simulink model "E010A5_R3_E1_event_queue_alloc_40A_1A_20260701_085331"  (R2024b)
settings: Solver=VariableStepAuto  StartTime=0.0  StopTime=0.54e-3  MaxStep=5e-9  RelTol=1e-3
undefined symbols (not defined in the file): A_init, A_lower, A_upper, Cout, DCR_L1, DCR_L2, DCR_L3, DCR_L4, E010_AreaBleed_Enable, E010_AreaHold_Enable, E010_AreaHold_Time, E010_PulseInhibit_Count, E010_PulseInhibit_Enable, E010_PulseInhibit_Time, E010_Reentry_Band_Down, E010_ReentryGuard_Enable, E010_TonTrunc_Enable, E010_Vref, E010A5_DeltaI_Drop_Threshold_High, E010A5_IL_Sense_Gain1, E010A5_IL_Sense_Gain2, E010A5_IL_Sense_Gain3, E010A5_IL_Sense_Gain4, E010A5_R3_AreaIntReentryTarget, E010A5_R3_AreaIntRestoreRate, E010A5_R3_AreaQueueCouplingEnable, E010A5_R3_EventQueue_Enable, E010A5_R3_FirstTonLimit, E010A5_R3_QueueMaxDepth, E010A5_R3_QueueReleaseMaxPerWindow, E010A5_R3_QueueReleaseMinSpacing, E010A5_R3_QueueSpacingEnable, E010A5_R3_TonBudget, E010A5_R3_TonBudgetWindow, E010A5_R3_TonMinMeaningful, E010A5_R3_TonRampMax, E010A5_R3_TonRampStep, E010A5_R3_UndershootBudget, E010A5_R3_UpperReentryBand, E010A5_R3_VoltageWindowEnable, ESR_C, IdealIQCOT_Enable, IL_adc_counts_per_A, IL_pk_limit_adc_neg, IL_pk_limit_adc_pos, Iload_final, Iload_initial, Iph, Iqcot_enable, kappa_cmd, Kiqcot, Kvc_iqcot, L, Lambda0_iqcot, Lambda_m2, rho_cmd, Ri_iqcot, t_load_step, Tblank, Tdead ... (+17)
libraries: simulink x29, spsCurrentMeasurementLib x8, spsMosfetLib x8, spsSeriesRLCBranchLib x5, spsVoltageMeasurementLib x5, spsDCVoltageSourceLib x4, spsControlledCurrentSourceLib x1, spsGroundLib x1, spspowerguiLib x1
(part 2 of 2)

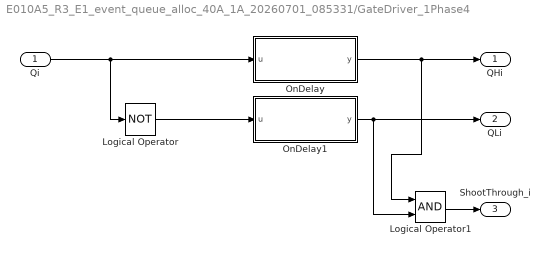
== system E010A5_R3_E1_event_queue_alloc_40A_1A_20260701_085331/GateDriver_1Phase4 ==
  Qi : Inport
  Logical Operator : Logic  Operator=NOT  AllPortsSameDT=off  OutDataTypeStr=boolean
  Logical Operator1 : Logic  AllPortsSameDT=off  OutDataTypeStr=boolean
  OnDelay : Subsystem
  OnDelay1 : Subsystem
  QHi : Outport
  QLi : Outport  Port=2
  ShootThrough_i : Outport  Port=3
  wires:
  Qi/1 -> Logical Operator/1, OnDelay/1(u)
  OnDelay/1(y) -> Logical Operator1/1, QHi/1
  Logical Operator/1 -> OnDelay1/1(u)
  OnDelay1/1(y) -> QLi/1, Logical Operator1/2
  Logical Operator1/1 -> ShootThrough_i/1

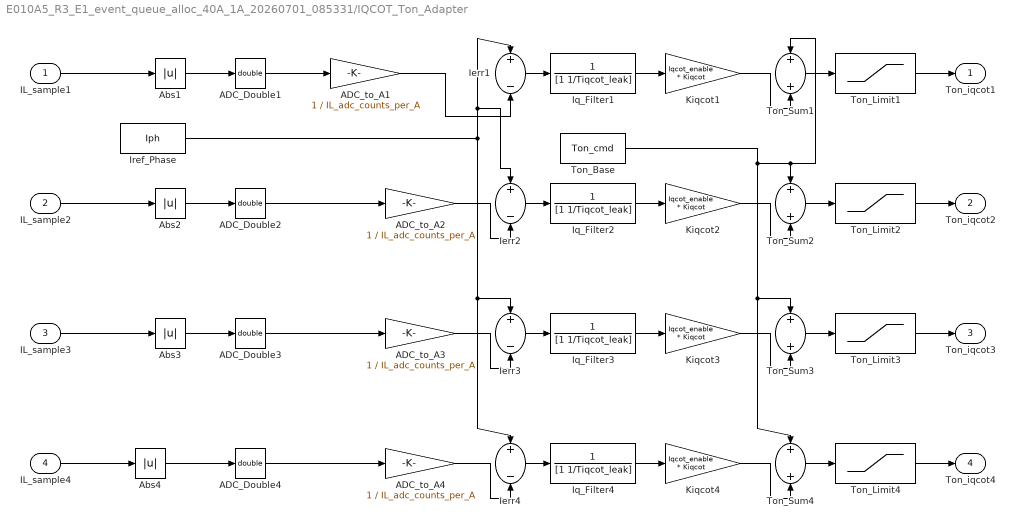
== system E010A5_R3_E1_event_queue_alloc_40A_1A_20260701_085331/IQCOT_Ton_Adapter ==
  IL_sample1 : Inport
  IL_sample2 : Inport  Port=2
  IL_sample3 : Inport  Port=3
  IL_sample4 : Inport  Port=4
  ADC_Double{1..4} (4 alike) : DataTypeConversion  OutDataTypeStr=double  SaturateOnIntegerOverflow=off  RndMeth=Floor
  ADC_to_A{1..4} (4 alike) : Gain  Gain=1 / IL_adc_counts_per_A  OutDataTypeStr=double
  Abs{1..4} (4 alike) : Abs  SaturateOnIntegerOverflow=off
  Ierr{1..4} (4 alike) : Sum  Inputs=+-
  Iq_Filter{1..4} (4 alike) : TransferFcn  Numerator=1  Denominator=[1 1/Tiqcot_leak]
  Iref_Phase : Constant  Value=Iph
  Kiqcot{1..4} (4 alike) : Gain  Gain=Iqcot_enable * Kiqcot
  Ton_Base : Constant  Value=Ton_cmd
  Ton_Limit{1..4} (4 alike) : Saturate  UpperLimit=Ton_iq_max  LowerLimit=Ton_iq_min
  Ton_Sum{1..4} (4 alike) : Sum
  Ton_iqcot1 : Outport
  Ton_iqcot2 : Outport  Port=2
  Ton_iqcot3 : Outport  Port=3
  Ton_iqcot4 : Outport  Port=4
  wires:
  IL_sample1/1 -> Abs1/1
  Abs1/1 -> ADC_Double1/1
  ADC_to_A1/1 -> Ierr1/2
  Iref_Phase/1 -> Ierr1/1, Ierr2/1, Ierr3/1, Ierr4/1
  Ierr1/1 -> Iq_Filter1/1
  Iq_Filter1/1 -> Kiqcot1/1
  Kiqcot1/1 -> Ton_Sum1/2
  Ton_Base/1 -> Ton_Sum3/1, Ton_Sum4/1, Ton_Sum1/1, Ton_Sum2/1
  Ton_Sum1/1 -> Ton_Limit1/1
  Ton_Limit1/1 -> Ton_iqcot1/1
  IL_sample2/1 -> Abs2/1
  Abs2/1 -> ADC_Double2/1
  ADC_to_A2/1 -> Ierr2/2
  Ierr2/1 -> Iq_Filter2/1
  Iq_Filter2/1 -> Kiqcot2/1
  Kiqcot2/1 -> Ton_Sum2/2
  Ton_Sum2/1 -> Ton_Limit2/1
  Ton_Limit2/1 -> Ton_iqcot2/1
  IL_sample3/1 -> Abs3/1
  Abs3/1 -> ADC_Double3/1
  ADC_to_A3/1 -> Ierr3/2
  Ierr3/1 -> Iq_Filter3/1
  Iq_Filter3/1 -> Kiqcot3/1
  Kiqcot3/1 -> Ton_Sum3/2
  Ton_Sum3/1 -> Ton_Limit3/1
  Ton_Limit3/1 -> Ton_iqcot3/1
  IL_sample4/1 -> Abs4/1
  Abs4/1 -> ADC_Double4/1
  ADC_to_A4/1 -> Ierr4/2
  Ierr4/1 -> Iq_Filter4/1
  Iq_Filter4/1 -> Kiqcot4/1
  Kiqcot4/1 -> Ton_Sum4/2
  Ton_Sum4/1 -> Ton_Limit4/1
  Ton_Limit4/1 -> Ton_iqcot4/1
  ADC_Double1/1 -> ADC_to_A1/1
  ADC_Double2/1 -> ADC_to_A2/1
  ADC_Double3/1 -> ADC_to_A3/1
  ADC_Double4/1 -> ADC_to_A4/1

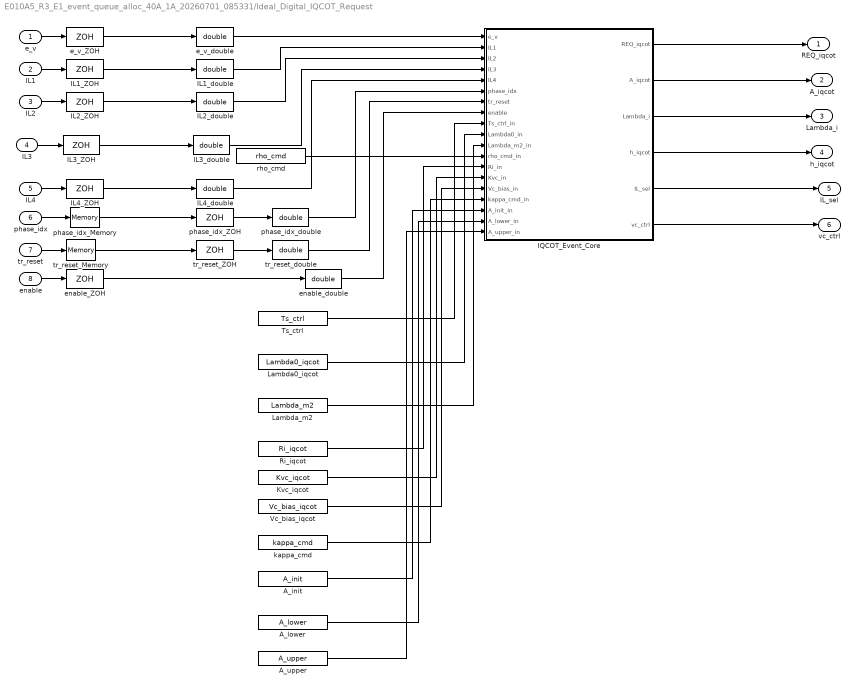
== system E010A5_R3_E1_event_queue_alloc_40A_1A_20260701_085331/Ideal_Digital_IQCOT_Request ==
  e_v : Inport
  IL1 : Inport  Port=2
  IL2 : Inport  Port=3
  IL3 : Inport  Port=4
  IL4 : Inport  Port=5
  phase_idx : Inport  Port=6
  tr_reset : Inport  Port=7
  enable : Inport  Port=8
  A_init : Constant  Value=A_init
  A_lower : Constant  Value=A_lower
  A_upper : Constant  Value=A_upper
  IL1_ZOH : ZeroOrderHold  SampleTime=Ts_ctrl
  IL1_double : DataTypeConversion  OutDataTypeStr=double  SaturateOnIntegerOverflow=off  RndMeth=Floor
  IL2_ZOH : ZeroOrderHold  SampleTime=Ts_ctrl
  IL2_double : DataTypeConversion  OutDataTypeStr=double  SaturateOnIntegerOverflow=off  RndMeth=Floor
  IL3_ZOH : ZeroOrderHold  SampleTime=Ts_ctrl
  IL3_double : DataTypeConversion  OutDataTypeStr=double  SaturateOnIntegerOverflow=off  RndMeth=Floor
  IL4_ZOH : ZeroOrderHold  SampleTime=Ts_ctrl
  IL4_double : DataTypeConversion  OutDataTypeStr=double  SaturateOnIntegerOverflow=off  RndMeth=Floor
  IQCOT_Event_Core : MATLAB Function  TreatAsAtomicUnit=on
  Kvc_iqcot : Constant  Value=Kvc_iqcot
  Lambda0_iqcot : Constant  Value=Lambda0_iqcot
  Lambda_m2 : Constant  Value=Lambda_m2
  Ri_iqcot : Constant  Value=Ri_iqcot
  Ts_ctrl : Constant  Value=Ts_ctrl
  Vc_bias_iqcot : Constant  Value=Vc_bias_iqcot
  e_v_ZOH : ZeroOrderHold  SampleTime=Ts_ctrl
  e_v_double : DataTypeConversion  OutDataTypeStr=double  SaturateOnIntegerOverflow=off  RndMeth=Floor
  enable_ZOH : ZeroOrderHold  SampleTime=Ts_ctrl
  enable_double : DataTypeConversion  OutDataTypeStr=double  SaturateOnIntegerOverflow=off  RndMeth=Floor
  kappa_cmd : Constant  Value=kappa_cmd
  phase_idx_Memory : Memory
  phase_idx_ZOH : ZeroOrderHold  SampleTime=Ts_ctrl
  phase_idx_double : DataTypeConversion  OutDataTypeStr=double  SaturateOnIntegerOverflow=off  RndMeth=Floor
  rho_cmd : Constant  Value=rho_cmd
  tr_reset_Memory : Memory
  tr_reset_ZOH : ZeroOrderHold  SampleTime=Ts_ctrl
  tr_reset_double : DataTypeConversion  OutDataTypeStr=double  SaturateOnIntegerOverflow=off  RndMeth=Floor
  REQ_iqcot : Outport
  A_iqcot : Outport  Port=2
  Lambda_i : Outport  Port=3
  h_iqcot : Outport  Port=4
  IL_sel : Outport  Port=5
  vc_ctrl : Outport  Port=6
  wires:
  e_v/1 -> e_v_ZOH/1
  e_v_ZOH/1 -> e_v_double/1
  IL1/1 -> IL1_ZOH/1
  IL1_ZOH/1 -> IL1_double/1
  IL2/1 -> IL2_ZOH/1
  IL2_ZOH/1 -> IL2_double/1
  IL3/1 -> IL3_ZOH/1
  IL3_ZOH/1 -> IL3_double/1
  IL4/1 -> IL4_ZOH/1
  IL4_ZOH/1 -> IL4_double/1
  phase_idx/1 -> phase_idx_Memory/1
  phase_idx_Memory/1 -> phase_idx_ZOH/1
  phase_idx_ZOH/1 -> phase_idx_double/1
  tr_reset/1 -> tr_reset_Memory/1
  tr_reset_Memory/1 -> tr_reset_ZOH/1
  tr_reset_ZOH/1 -> tr_reset_double/1
  enable/1 -> enable_ZOH/1
  enable_ZOH/1 -> enable_double/1
  e_v_double/1 -> IQCOT_Event_Core/1(e_v)
  IL1_double/1 -> IQCOT_Event_Core/2(IL1)
  IL2_double/1 -> IQCOT_Event_Core/3(IL2)
  IL3_double/1 -> IQCOT_Event_Core/4(IL3)
  IL4_double/1 -> IQCOT_Event_Core/5(IL4)
  phase_idx_double/1 -> IQCOT_Event_Core/6(phase_idx)
  tr_reset_double/1 -> IQCOT_Event_Core/7(tr_reset)
  enable_double/1 -> IQCOT_Event_Core/8(enable)
  Ts_ctrl/1 -> IQCOT_Event_Core/9(Ts_ctrl_in)
  Lambda0_iqcot/1 -> IQCOT_Event_Core/10(Lambda0_in)
  Lambda_m2/1 -> IQCOT_Event_Core/11(Lambda_m2_in)
  rho_cmd/1 -> IQCOT_Event_Core/12(rho_cmd_in)
  Ri_iqcot/1 -> IQCOT_Event_Core/13(Ri_in)
  Kvc_iqcot/1 -> IQCOT_Event_Core/14(Kvc_in)
  Vc_bias_iqcot/1 -> IQCOT_Event_Core/15(Vc_bias_in)
  kappa_cmd/1 -> IQCOT_Event_Core/16(kappa_cmd_in)
  A_init/1 -> IQCOT_Event_Core/17(A_init_in)
  A_lower/1 -> IQCOT_Event_Core/18(A_lower_in)
  A_upper/1 -> IQCOT_Event_Core/19(A_upper_in)
  IQCOT_Event_Core/1(REQ_iqcot) -> REQ_iqcot/1
  IQCOT_Event_Core/2(A_iqcot) -> A_iqcot/1
  IQCOT_Event_Core/3(Lambda_i) -> Lambda_i/1
  IQCOT_Event_Core/4(h_iqcot) -> h_iqcot/1
  IQCOT_Event_Core/5(IL_sel) -> IL_sel/1
  IQCOT_Event_Core/6(vc_ctrl) -> vc_ctrl/1

== system E010A5_R3_E1_event_queue_alloc_40A_1A_20260701_085331/OnDelay ==
  u : Inport
  Compare To Constant : simulink/Logic and Bit Operations/Compare To Constant  relop=>=  const=Tdead  OutDataTypeStr=boolean
  Data Type Conversion : DataTypeConversion  OutDataTypeStr=double  SaturateOnIntegerOverflow=off  RndMeth=Floor
  Integrator : Integrator  ExternalReset=level
  Logical Operator : Logic  Operator=NOT  AllPortsSameDT=off  OutDataTypeStr=boolean
  y : Outport
  wires:
  u/1 -> Data Type Conversion/1, Logical Operator/1
  Logical Operator/1 -> Integrator/2
  Data Type Conversion/1 -> Integrator/1
  Integrator/1 -> Compare To Constant/1
  Compare To Constant/1 -> y/1

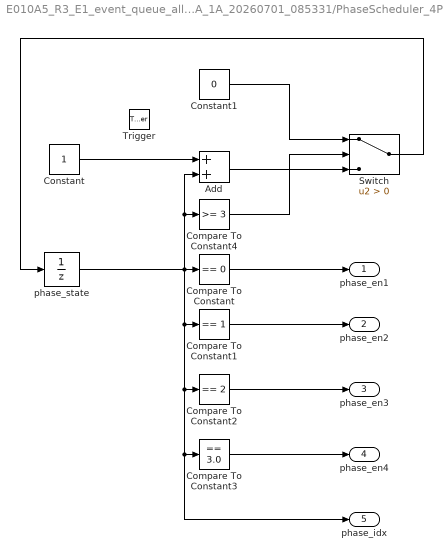
== system E010A5_R3_E1_event_queue_alloc_40A_1A_20260701_085331/PhaseScheduler_4Phase ==
  Trigger : TriggerPort  VariantControl=(inherit)
  Add : Sum
  Compare To Constant : simulink/Logic and Bit Operations/Compare To Constant  relop===  const=0  OutDataTypeStr=boolean
  Compare To Constant1 : simulink/Logic and Bit Operations/Compare To Constant  relop===  const=1  OutDataTypeStr=boolean
  Compare To Constant2 : simulink/Logic and Bit Operations/Compare To Constant  relop===  const=2  OutDataTypeStr=boolean
  Compare To Constant3 : simulink/Logic and Bit Operations/Compare To Constant  relop===  const=3.0  OutDataTypeStr=boolean
  Compare To Constant4 : simulink/Logic and Bit Operations/Compare To Constant  relop=>=  const=3  OutDataTypeStr=boolean
  Constant : Constant
  Constant1 : Constant  Value=0
  Switch : Switch  Criteria=u2 > Threshold  SaturateOnIntegerOverflow=off  InputSameDT=off
  phase_state : UnitDelay  SampleTime=-1  HasFrameUpgradeWarning=on
  phase_en1 : Outport
  phase_en2 : Outport  Port=2
  phase_en3 : Outport  Port=3
  phase_en4 : Outport  Port=4
  phase_idx : Outport  Port=5
  wires:
  phase_state/1 -> phase_idx/1, Compare To Constant3/1, Compare To Constant2/1, Compare To Constant1/1, Compare To Constant/1, Compare To Constant4/1, Add/2
  Compare To Constant/1 -> phase_en1/1
  Compare To Constant1/1 -> phase_en2/1
  Compare To Constant2/1 -> phase_en3/1
  Compare To Constant3/1 -> phase_en4/1
  Constant/1 -> Add/1
  Add/1 -> Switch/3
  Compare To Constant4/1 -> Switch/2
  Constant1/1 -> Switch/1
  Switch/1 -> phase_state/1

== system E010A5_R3_E1_event_queue_alloc_40A_1A_20260701_085331/GateDriver_1Phase1/OnDelay ==
  u : Inport
  Compare To Constant : simulink/Logic and Bit Operations/Compare To Constant  relop=>=  const=Tdead  OutDataTypeStr=boolean
  Data Type Conversion : DataTypeConversion  OutDataTypeStr=double  SaturateOnIntegerOverflow=off  RndMeth=Floor
  Integrator : Integrator  ExternalReset=level
  Logical Operator : Logic  Operator=NOT  AllPortsSameDT=off  OutDataTypeStr=boolean
  y : Outport
  wires:
  u/1 -> Data Type Conversion/1, Logical Operator/1
  Logical Operator/1 -> Integrator/2
  Data Type Conversion/1 -> Integrator/1
  Integrator/1 -> Compare To Constant/1
  Compare To Constant/1 -> y/1

== system E010A5_R3_E1_event_queue_alloc_40A_1A_20260701_085331/GateDriver_1Phase1/OnDelay1 ==
  u : Inport
  Compare To Constant : simulink/Logic and Bit Operations/Compare To Constant  relop=>=  const=Tdead  OutDataTypeStr=boolean
  Data Type Conversion : DataTypeConversion  OutDataTypeStr=double  SaturateOnIntegerOverflow=off  RndMeth=Floor
  Integrator : Integrator  ExternalReset=level
  Logical Operator : Logic  Operator=NOT  AllPortsSameDT=off  OutDataTypeStr=boolean
  y : Outport
  wires:
  u/1 -> Data Type Conversion/1, Logical Operator/1
  Logical Operator/1 -> Integrator/2
  Data Type Conversion/1 -> Integrator/1
  Integrator/1 -> Compare To Constant/1
  Compare To Constant/1 -> y/1

== system E010A5_R3_E1_event_queue_alloc_40A_1A_20260701_085331/GateDriver_1Phase2/OnDelay ==
  u : Inport
  Compare To Constant : simulink/Logic and Bit Operations/Compare To Constant  relop=>=  const=Tdead  OutDataTypeStr=boolean
  Data Type Conversion : DataTypeConversion  OutDataTypeStr=double  SaturateOnIntegerOverflow=off  RndMeth=Floor
  Integrator : Integrator  ExternalReset=level
  Logical Operator : Logic  Operator=NOT  AllPortsSameDT=off  OutDataTypeStr=boolean
  y : Outport
  wires:
  u/1 -> Data Type Conversion/1, Logical Operator/1
  Logical Operator/1 -> Integrator/2
  Data Type Conversion/1 -> Integrator/1
  Integrator/1 -> Compare To Constant/1
  Compare To Constant/1 -> y/1

== system E010A5_R3_E1_event_queue_alloc_40A_1A_20260701_085331/GateDriver_1Phase2/OnDelay1 ==
  u : Inport
  Compare To Constant : simulink/Logic and Bit Operations/Compare To Constant  relop=>=  const=Tdead  OutDataTypeStr=boolean
  Data Type Conversion : DataTypeConversion  OutDataTypeStr=double  SaturateOnIntegerOverflow=off  RndMeth=Floor
  Integrator : Integrator  ExternalReset=level
  Logical Operator : Logic  Operator=NOT  AllPortsSameDT=off  OutDataTypeStr=boolean
  y : Outport
  wires:
  u/1 -> Data Type Conversion/1, Logical Operator/1
  Logical Operator/1 -> Integrator/2
  Data Type Conversion/1 -> Integrator/1
  Integrator/1 -> Compare To Constant/1
  Compare To Constant/1 -> y/1

== system E010A5_R3_E1_event_queue_alloc_40A_1A_20260701_085331/GateDriver_1Phase3/OnDelay ==
  u : Inport
  Compare To Constant : simulink/Logic and Bit Operations/Compare To Constant  relop=>=  const=Tdead  OutDataTypeStr=boolean
  Data Type Conversion : DataTypeConversion  OutDataTypeStr=double  SaturateOnIntegerOverflow=off  RndMeth=Floor
  Integrator : Integrator  ExternalReset=level
  Logical Operator : Logic  Operator=NOT  AllPortsSameDT=off  OutDataTypeStr=boolean
  y : Outport
  wires:
  u/1 -> Data Type Conversion/1, Logical Operator/1
  Logical Operator/1 -> Integrator/2
  Data Type Conversion/1 -> Integrator/1
  Integrator/1 -> Compare To Constant/1
  Compare To Constant/1 -> y/1

== system E010A5_R3_E1_event_queue_alloc_40A_1A_20260701_085331/GateDriver_1Phase3/OnDelay1 ==
  u : Inport
  Compare To Constant : simulink/Logic and Bit Operations/Compare To Constant  relop=>=  const=Tdead  OutDataTypeStr=boolean
  Data Type Conversion : DataTypeConversion  OutDataTypeStr=double  SaturateOnIntegerOverflow=off  RndMeth=Floor
  Integrator : Integrator  ExternalReset=level
  Logical Operator : Logic  Operator=NOT  AllPortsSameDT=off  OutDataTypeStr=boolean
  y : Outport
  wires:
  u/1 -> Data Type Conversion/1, Logical Operator/1
  Logical Operator/1 -> Integrator/2
  Data Type Conversion/1 -> Integrator/1
  Integrator/1 -> Compare To Constant/1
  Compare To Constant/1 -> y/1

== system E010A5_R3_E1_event_queue_alloc_40A_1A_20260701_085331/GateDriver_1Phase4/OnDelay ==
  u : Inport
  Compare To Constant : simulink/Logic and Bit Operations/Compare To Constant  relop=>=  const=Tdead  OutDataTypeStr=boolean
  Data Type Conversion : DataTypeConversion  OutDataTypeStr=double  SaturateOnIntegerOverflow=off  RndMeth=Floor
  Integrator : Integrator  ExternalReset=level
  Logical Operator : Logic  Operator=NOT  AllPortsSameDT=off  OutDataTypeStr=boolean
  y : Outport
  wires:
  u/1 -> Data Type Conversion/1, Logical Operator/1
  Logical Operator/1 -> Integrator/2
  Data Type Conversion/1 -> Integrator/1
  Integrator/1 -> Compare To Constant/1
  Compare To Constant/1 -> y/1

== system E010A5_R3_E1_event_queue_alloc_40A_1A_20260701_085331/GateDriver_1Phase4/OnDelay1 ==
  u : Inport
  Compare To Constant : simulink/Logic and Bit Operations/Compare To Constant  relop=>=  const=Tdead  OutDataTypeStr=boolean
  Data Type Conversion : DataTypeConversion  OutDataTypeStr=double  SaturateOnIntegerOverflow=off  RndMeth=Floor
  Integrator : Integrator  ExternalReset=level
  Logical Operator : Logic  Operator=NOT  AllPortsSameDT=off  OutDataTypeStr=boolean
  y : Outport
  wires:
  u/1 -> Data Type Conversion/1, Logical Operator/1
  Logical Operator/1 -> Integrator/2
  Data Type Conversion/1 -> Integrator/1
  Integrator/1 -> Compare To Constant/1
  Compare To Constant/1 -> y/1

== matlab function E010A5_R3_E1_event_queue_alloc_40A_1A_20260701_085331/E010A5_CurrentLimitHit ==
  data: u1 input boolean size=1; y output double size=1; u2 input boolean size=1; u3 input boolean size=1; u4 input boolean size=1
function y = any_four(u1,u2,u3,u4)
%#codegen
y = double((u1 > 0.5) || (u2 > 0.5) || (u3 > 0.5) || (u4 > 0.5));

== matlab function E010A5_R3_E1_event_queue_alloc_40A_1A_20260701_085331/E010A5_TonTrunc1 ==
  data: ton_in input double size=1; ton_out output double size=1; t input double size=1; t_step input double size=1; t_window input double size=1; t_min input double size=1; enable input double size=1; trunc_active output double size=1; ton_saved output double size=1
function [ton_out,trunc_active,ton_saved] = ton_trunc(ton_in,t,t_step,t_window,t_min,enable)
%#codegen
active = (enable > 0.5) && (t >= t_step) && (t <= (t_step + t_window));
if active
    ton_out = min(ton_in, t_min);
else
    ton_out = ton_in;
end
trunc_active = double(active);
ton_saved = max(ton_in - ton_out, 0.0);

== matlab function E010A5_R3_E1_event_queue_alloc_40A_1A_20260701_085331/E010A5_TonTrunc2 ==
  data: ton_in input double size=1; ton_out output double size=1; t input double size=1; t_step input double size=1; t_window input double size=1; t_min input double size=1; enable input double size=1; trunc_active output double size=1; ton_saved output double size=1
function [ton_out,trunc_active,ton_saved] = ton_trunc(ton_in,t,t_step,t_window,t_min,enable)
%#codegen
active = (enable > 0.5) && (t >= t_step) && (t <= (t_step + t_window));
if active
    ton_out = min(ton_in, t_min);
else
    ton_out = ton_in;
end
trunc_active = double(active);
ton_saved = max(ton_in - ton_out, 0.0);

== matlab function E010A5_R3_E1_event_queue_alloc_40A_1A_20260701_085331/E010A5_TonTrunc3 ==
  data: ton_in input double size=1; ton_out output double size=1; t input double size=1; t_step input double size=1; t_window input double size=1; t_min input double size=1; enable input double size=1; trunc_active output double size=1; ton_saved output double size=1
function [ton_out,trunc_active,ton_saved] = ton_trunc(ton_in,t,t_step,t_window,t_min,enable)
%#codegen
active = (enable > 0.5) && (t >= t_step) && (t <= (t_step + t_window));
if active
    ton_out = min(ton_in, t_min);
else
    ton_out = ton_in;
end
trunc_active = double(active);
ton_saved = max(ton_in - ton_out, 0.0);

== matlab function E010A5_R3_E1_event_queue_alloc_40A_1A_20260701_085331/E010A5_TonTrunc4 ==
  data: ton_in input double size=1; ton_out output double size=1; t input double size=1; t_step input double size=1; t_window input double size=1; t_min input double size=1; enable input double size=1; trunc_active output double size=1; ton_saved output double size=1
function [ton_out,trunc_active,ton_saved] = ton_trunc(ton_in,t,t_step,t_window,t_min,enable)
%#codegen
active = (enable > 0.5) && (t >= t_step) && (t <= (t_step + t_window));
if active
    ton_out = min(ton_in, t_min);
else
    ton_out = ton_in;
end
trunc_active = double(active);
ton_saved = max(ton_in - ton_out, 0.0);

== matlab function E010A5_R3_E1_event_queue_alloc_40A_1A_20260701_085331/E010A5_PulseInhibitState ==
  data: u1 input boolean size=1; y output double size=1; u2 input boolean size=1; u3 input boolean size=1; u4 input boolean size=1
function y = any_four(u1,u2,u3,u4)
%#codegen
y = double((u1 > 0.5) || (u2 > 0.5) || (u3 > 0.5) || (u4 > 0.5));

== matlab function E010A5_R3_E1_event_queue_alloc_40A_1A_20260701_085331/E010A5_PulseInhibit1 ==
  data: tr_in input boolean size=1; tr_out output boolean size=1; t input double size=1; t_step input double size=1; t_window input double size=1; count_max input double size=1; enable input double size=1; vout input double size=1; vref input double size=1; reentry_band input double size=1; guard_enable input double size=1; inhibit_active output boolean size=1; inhibit_count output double size=1
function [tr_out,inhibit_active,inhibit_count] = pulse_inhibit(tr_in,t,t_step,t_window,count_max,enable,vout,vref,reentry_band,guard_enable)
%#codegen
is_high = logical(tr_in);
in_window = (enable > 0.5) && (t >= t_step) && (t <= (t_step + t_window));
guard_ok = (guard_enable <= 0.5) || (vout >= (vref + reentry_band));
inhibit_active = is_high && in_window && (count_max > 0.0) && guard_ok;
if inhibit_active
    tr_out = false;
else
    tr_out = tr_in;
end
inhibit_count = double(inhibit_active);

== matlab function E010A5_R3_E1_event_queue_alloc_40A_1A_20260701_085331/E010A5_PulseInhibit2 ==
  data: tr_in input boolean size=1; tr_out output boolean size=1; t input double size=1; t_step input double size=1; t_window input double size=1; count_max input double size=1; enable input double size=1; vout input double size=1; vref input double size=1; reentry_band input double size=1; guard_enable input double size=1; inhibit_active output boolean size=1; inhibit_count output double size=1
function [tr_out,inhibit_active,inhibit_count] = pulse_inhibit(tr_in,t,t_step,t_window,count_max,enable,vout,vref,reentry_band,guard_enable)
%#codegen
is_high = logical(tr_in);
in_window = (enable > 0.5) && (t >= t_step) && (t <= (t_step + t_window));
guard_ok = (guard_enable <= 0.5) || (vout >= (vref + reentry_band));
inhibit_active = is_high && in_window && (count_max > 0.0) && guard_ok;
if inhibit_active
    tr_out = false;
else
    tr_out = tr_in;
end
inhibit_count = double(inhibit_active);

== matlab function E010A5_R3_E1_event_queue_alloc_40A_1A_20260701_085331/E010A5_PulseInhibit3 ==
  data: tr_in input boolean size=1; tr_out output boolean size=1; t input double size=1; t_step input double size=1; t_window input double size=1; count_max input double size=1; enable input double size=1; vout input double size=1; vref input double size=1; reentry_band input double size=1; guard_enable input double size=1; inhibit_active output boolean size=1; inhibit_count output double size=1
function [tr_out,inhibit_active,inhibit_count] = pulse_inhibit(tr_in,t,t_step,t_window,count_max,enable,vout,vref,reentry_band,guard_enable)
%#codegen
is_high = logical(tr_in);
in_window = (enable > 0.5) && (t >= t_step) && (t <= (t_step + t_window));
guard_ok = (guard_enable <= 0.5) || (vout >= (vref + reentry_band));
inhibit_active = is_high && in_window && (count_max > 0.0) && guard_ok;
if inhibit_active
    tr_out = false;
else
    tr_out = tr_in;
end
inhibit_count = double(inhibit_active);

== matlab function E010A5_R3_E1_event_queue_alloc_40A_1A_20260701_085331/E010A5_PulseInhibit4 ==
  data: tr_in input boolean size=1; tr_out output boolean size=1; t input double size=1; t_step input double size=1; t_window input double size=1; count_max input double size=1; enable input double size=1; vout input double size=1; vref input double size=1; reentry_band input double size=1; guard_enable input double size=1; inhibit_active output boolean size=1; inhibit_count output double size=1
function [tr_out,inhibit_active,inhibit_count] = pulse_inhibit(tr_in,t,t_step,t_window,count_max,enable,vout,vref,reentry_band,guard_enable)
%#codegen
is_high = logical(tr_in);
in_window = (enable > 0.5) && (t >= t_step) && (t <= (t_step + t_window));
guard_ok = (guard_enable <= 0.5) || (vout >= (vref + reentry_band));
inhibit_active = is_high && in_window && (count_max > 0.0) && guard_ok;
if inhibit_active
    tr_out = false;
else
    tr_out = tr_in;
end
inhibit_count = double(inhibit_active);

== matlab function E010A5_R3_E1_event_queue_alloc_40A_1A_20260701_085331/E010A5_AreaHold_EnableProjection ==
  data: enable_in input double size=1; enable_out output double size=1; t input double size=1; t_step input double size=1; t_hold input double size=1; hold_enable input double size=1; vout input double size=1; vref input double size=1; reentry_band input double size=1; bleed_enable input double size=1; hold_state output double size=1; hold_count output double size=1; reset_count output double size=1; bleed_count output double size=1; reentry_state output double size=1
function [enable_out,hold_state,hold_count,reset_count,bleed_count,reentry_state] = area_hold_enable(enable_in,t,t_step,t_hold,hold_enable,vout,vref,reentry_band,bleed_enable)
%#codegen
persistent was_hold reset_seen
if isempty(was_hold)
    was_hold = false;
end
if isempty(reset_seen)
    reset_seen = 0.0;
end
if t < t_step
    was_hold = false;
    reset_seen = 0.0;
end
in_window = (hold_enable > 0.5) && (t >= t_step) && (t <= (t_step + t_hold));
release_not_safe = vout >= (vref + reentry_band);
hold = in_window && release_not_safe;
enable_out = double(enable_in > 0.5);
if hold
    enable_out = 0.0;
end
hold_state = double(hold);
hold_count = double(hold);
bleed_count = double(hold && (bleed_enable > 0.5));
release_edge = (~hold) && was_hold;
if release_edge
    reset_seen = reset_seen + 1.0;
end
reset_count = reset_seen;
reentry_state = double((hold_enable > 0.5) && (t > t_step) && ~hold);
was_hold = hold;

== matlab function E010A5_R3_E1_event_queue_alloc_40A_1A_20260701_085331/E010A5_R3_EventQueueAllocator ==
  data: req1 input boolean size=1; req1o output boolean size=1; req2 input boolean size=1; req3 input boolean size=1; req4 input boolean size=1; ton1 input double size=1; ton2 input double size=1; ton3 input double size=1; ton4 input double size=1; t input double size=1; t_step input double size=1; enable input double size=1; queue_max_depth input double size=1; min_spacing input double size=1; max_per_window input double size=1; spacing_enable input double size=1; budget_window input double size=1; ton_budget input double size=1; ton_min input double size=1; first_limit input double size=1; ramp_step input double size=1; max_ton input double size=1; area_enable input double size=1; area_int input double size=1; area_target input double size=1; area_restore_rate input double size=1; voltage_enable input double size=1; vout input double size=1; vref input double size=1; upper_band input double size=1; undershoot_budget input double size=1; req2o output boolean size=1; req3o output boolean size=1; req4o output boolean size=1; ton1o output double size=1; ton2o output double size=1; ton3o output double size=1; ton4o output double size=1; d1 output boolean size=1; d2 output boolean size=1; d3 output boolean size=1; d4 output boolean size=1; pending output double size=1; queue_depth output double size=1; queue_age_us output double size=1; queue_phase_id output double size=1; queue_reason output double size=1; queue_release_time output double size=1; queue_energy_budget_ns output double size=1; queue_release_count output double size=1; queue_reject_count output double size=1; queue_reject_reason output double size=1; Ton_requested_ns output double size=1; Ton_allocated_ns output double size=1; Ton_budget_remaining_ns output double size=1; Ton_allocation_reason output double size=1; reentry_Ton_budget_used_ns output double size=1; reentry_Ton_budget_violation output double size=1; area_int_capture_at_drop output double size=1; area_int_reentry_target output double size=1; area_int_restore_usage output double size=1; area_int_queue_coupling_usage output double size=1; area_int_queue_coupling_state output double size=1; area_int_restore_state output double size=1; event_queue_state output double size=1; energy_allocation_state output double size=1; controlled_reentry_active output double size=1; actual_inter_pulse_spacing output double size=1; burst_pulse_count_after_reentry output double size=1
function [req1o,req2o,req3o,req4o,ton1o,ton2o,ton3o,ton4o,d1,d2,d3,d4,pending,queue_depth,queue_age_us,queue_phase_id,queue_reason,queue_release_time,queue_energy_budget_ns,queue_release_count,queue_reject_count,queue_reject_reason,Ton_requested_ns,Ton_allocated_ns,Ton_budget_remaining_ns,Ton_allocation_reason,reentry_Ton_budget_used_ns,reentry_Ton_budget_violation,area_int_capture_at_drop,area_int_reentry_target,area_int_restore_usage,area_int_queue_coupling_usage,area_int_queue_coupling_state,area_int_restore_state,event_queue_state,energy_allocation_state,controlled_reentry_active,actual_inter_pulse_spacing,burst_pulse_count_after_reentry] = r3_event_queue(req1,req2,req3,req4,ton1,ton2,ton3,ton4,t,t_step,enable,queue_max_depth,min_spacing,max_per_window,spacing_enable,budget_window,ton_budget,ton_min,first_limit,ramp_step,max_ton,area_enable,area_int,area_target,area_restore_rate,voltage_enable,vout,vref,upper_band,undershoot_budget)
%#codegen
persistent prev_req q_phase q_ton q_time q_reason q_depth used first_time
persistent last_release release_window_start release_count_total reject_count_total
persistent capture_set area_capture last_req_ns last_alloc_ns last_reason last_spacing
persistent hold_phase hold_until hold_ton last_release_rel_us
if isempty(prev_req)
    prev_req = [false,false,false,false];
    q_phase = zeros(1,4);
    q_ton = zeros(1,4);
    q_time = zeros(1,4);
    q_reason = zeros(1,4);
    q_depth = 0.0;
    used = 0.0;
    first_time = -1.0;
    last_release = -1.0;
    release_window_start = -1.0;
    release_count_total = 0.0;
    reject_count_total = 0.0;
    capture_set = false;
    area_capture = 0.0;
    last_req_ns = 0.0;
    last_alloc_ns = 0.0;
    last_reason = 0.0;
    last_spacing = 0.0;
    hold_phase = 0.0;
    hold_until = -1.0;
    hold_ton = 0.0;
    last_release_rel_us = 0.0;
end
if t < t_step
    prev_req = [false,false,false,false];
    q_phase(:) = 0.0;
    q_ton(:) = 0.0;
    q_time(:) = 0.0;
    q_reason(:) = 0.0;
    q_depth = 0.0;
    used = 0.0;
    first_time = -1.0;
    last_release = -1.0;
    release_window_start = -1.0;
    release_count_total = 0.0;
    reject_count_total = 0.0;
    capture_set = false;
    area_capture = 0.0;
    last_req_ns = 0.0;
    last_alloc_ns = 0.0;
    last_reason = 0.0;
    last_spacing = 0.0;
    hold_phase = 0.0;
    hold_until = -1.0;
    hold_ton = 0.0;
    last_release_rel_us = 0.0;
end
req = [req1,req2,req3,req4] > 0.5;
rise = req & ~prev_req;
tons = [ton1,ton2,ton3,ton4];
req_out = [false,false,false,false];
defer = [false,false,false,false];
ton_out = tons;
active = (enable > 0.5) && (t >= t_step);
if active && ~capture_set
    area_capture = area_int;
    capture_set = true;
end
if active && (first_time < 0.0) && any(rise)
    first_time = t;
    release_window_start = t;
end
if first_time >= 0.0
    age = max(t - first_time, 0.0);
else
    age = 0.0;
end
in_budget_window = active && (first_time >= 0.0) && (age <= max(budget_window, 0.0));
if (release_window_start < 0.0) || ((t - release_window_start) > max(budget_window, 1.0e-12))
    release_window_start = t;
    release_count_total = 0.0;
end
budget_remaining = max(ton_budget - used, 0.0);
if ~in_budget_window
    budget_remaining = max(max_ton, ton_min);
end
ramp_limit = min(max_ton, max(first_limit, first_limit + release_count_total * max(ramp_step, 0.0)));
spacing_ok = (spacing_enable <= 0.5) || (last_release < 0.0) || ((t - last_release) >= max(min_spacing, 0.0));
window_ok = (spacing_enable <= 0.5) || (release_count_total < max(max_per_window, 1.0));
voltage_ok = (voltage_enable <= 0.5) || ((vout <= vref + max(upper_band, 0.0)) && (vout >= vref - max(undershoot_budget, 0.0)));
area_tol = max(abs(area_target), 1.0e-9) + 5.0e-7;
area_ok = (area_enable <= 0.5) || (abs(area_int - area_target) <= area_tol);
budget_ok = budget_remaining >= max(ton_min, 0.0);
release_ok = active && spacing_ok && window_ok && voltage_ok && area_ok && budget_ok;
holding = (hold_phase >= 1.0) && (t < hold_until);
if holding
    hp = min(max(round(hold_phase), 1), 4);
    req_out(hp) = true;
    ton_out(hp) = hold_ton;
end
released_this_step = false;
if active && ~holding && (q_depth > 0.5) && release_ok
    qp = min(max(round(q_phase(1)), 1), 4);
    requested = max(q_ton(1), 0.0);
    allocated = min([requested, budget_remaining, ramp_limit]);
    last_req_ns = 1.0e9 * requested;
    if allocated >= max(ton_min, 0.0)
        req_out(qp) = true;
        ton_out(qp) = allocated;
        hold_phase = qp;
        hold_until = t + 25.0e-9;
        hold_ton = allocated;
        used = used + double(in_budget_window) * allocated;
        if last_release >= 0.0
            last_spacing = t - last_release;
        else
            last_spacing = 0.0;
        end
        last_release = t;
        last_release_rel_us = 1.0e6 * (t - t_step);
        release_count_total = release_count_total + 1.0;
        last_alloc_ns = 1.0e9 * allocated;
        last_reason = 2.0;
        released_this_step = true;
        for k = 1:3
            q_phase(k) = q_phase(k+1);
            q_ton(k) = q_ton(k+1);
            q_time(k) = q_time(k+1);
            q_reason(k) = q_reason(k+1);
        end
        q_phase(4) = 0.0; q_ton(4) = 0.0; q_time(4) = 0.0; q_reason(4) = 0.0;
        q_depth = max(q_depth - 1.0, 0.0);
    else
        last_reason = 4.0;
    end
end
hold_pass_through = active && (in_budget_window || q_depth > 0.5 || spacing_enable > 0.5 || area_enable > 0.5 || voltage_enable > 0.5);
for idx = 1:4
    if rise(idx)
        requested = max(tons(idx), 0.0);
        last_req_ns = 1.0e9 * requested;
        should_control = hold_pass_through;
        if should_control
            can_try_now = (q_depth < 0.5) && ~holding && ~released_this_step && release_ok;
            allocated = min([requested, budget_remaining, ramp_limit]);
            if can_try_now && (allocated >= max(ton_min, 0.0))
                req_out(idx) = true;
                ton_out(idx) = allocated;
                hold_phase = idx;
                hold_until = t + 25.0e-9;
                hold_ton = allocated;
                used = used + double(in_budget_window) * allocated;
                if last_release >= 0.0
                    last_spacing = t - last_release;
                else
                    last_spacing = 0.0;
                end
                last_release = t;
                last_release_rel_us = 1.0e6 * (t - t_step);
                release_count_total = release_count_total + 1.0;
                last_alloc_ns = 1.0e9 * allocated;
                last_reason = 1.0;
                released_this_step = true;
            else
                reason = 3.0;
                if ~budget_ok
                    reason = 4.0;
                elseif ~voltage_ok
                    reason = 5.0;
                elseif ~area_ok
                    reason = 6.0;
                elseif ~spacing_ok || ~window_ok
                    reason = 7.0;
                elseif allocated < max(ton_min, 0.0)
                    reason = 8.0;
                end
                if q_depth < min(max(queue_max_depth, 1.0), 4.0)
                    slot = min(max(round(q_depth + 1.0), 1), 4);
                    q_phase(slot) = idx;
                    q_ton(slot) = requested;
                    q_time(slot) = t;
                    q_reason(slot) = reason;
                    q_depth = q_depth + 1.0;
                    defer(idx) = true;
                    last_reason = reason;
                else
                    reject_count_total = reject_count_total + 1.0;
                    last_reason = 9.0;
                end
            end
        else
            req_out(idx) = true;
            ton_out(idx) = requested;
            last_alloc_ns = 1.0e9 * requested;
            last_reason = 10.0;
        end
    elseif ~hold_pass_through
        req_out(idx) = req(idx);
    end
end
pending = double(q_depth > 0.5);
if q_depth > 0.5
    queue_age_us = 1.0e6 * max(t - q_time(1), 0.0);
    queue_phase_id = q_phase(1);
    queue_reason = q_reason(1);
else
    queue_age_us = 0.0;
    queue_phase_id = 0.0;
    queue_reason = 0.0;
end
queue_release_time = last_release_rel_us;
queue_energy_budget_ns = 1.0e9 * budget_remaining;
queue_release_count = release_count_total;
queue_reject_count = reject_count_total;
queue_reject_reason = double(last_reason == 9.0) * 9.0;
Ton_requested_ns = last_req_ns;
Ton_allocated_ns = last_alloc_ns;
Ton_budget_remaining_ns = 1.0e9 * budget_remaining;
Ton_allocation_reason = last_reason;
reentry_Ton_budget_used_ns = 1.0e9 * used;
reentry_Ton_budget_violation = double(in_budget_window && (used > ton_budget + 1.0e-12));
area_int_capture_at_drop = area_capture;
area_int_reentry_target = area_target;
if area_enable > 0.5
    area_int_restore_usage = min(max(age * max(area_restore_rate, 0.0), 0.0), 1.0);
    area_int_queue_coupling_usage = double(q_depth > 0.5) * area_int_restore_usage;
    area_int_queue_coupling_state = 1.0 + double(~area_ok);
    area_int_restore_state = double(area_int_restore_usage > 0.0);
else
    area_int_restore_usage = 0.0;
    area_int_queue_coupling_usage = 0.0;
    area_int_queue_coupling_state = 0.0;
    area_int_restore_state = 0.0;
end
if ~active
    event_queue_state = 0.0;
elseif q_depth > 0.5
    event_queue_state = 2.0;
elseif released_this_step
    event_queue_state = 3.0;
else
    event_queue_state = 1.0;
end
if last_reason == 1.0 || last_reason == 2.0 || last_reason == 10.0
    energy_allocation_state = 1.0;
elseif last_reason == 4.0 || last_reason == 8.0
    energy_allocation_state = 3.0;
elseif last_reason == 0.0
    energy_allocation_state = 0.0;
else
    energy_allocation_state = 2.0;
end
controlled_reentry_active = double(active && (in_budget_window || q_depth > 0.5));
actual_inter_pulse_spacing = 1.0e6 * last_spacing;
burst_pulse_count_after_reentry = release_count_total;
req1o = req_out(1); req2o = req_out(2); req3o = req_out(3); req4o = req_out(4);
ton1o = ton_out(1); ton2o = ton_out(2); ton3o = ton_out(3); ton4o = ton_out(4);
d1 = defer(1); d2 = defer(2); d3 = defer(3); d4 = defer(4);
queue_depth = q_depth;
prev_req = req;
end

== matlab function E010A5_R3_E1_event_queue_alloc_40A_1A_20260701_085331/E010A5_REQRejectReason ==
  data: r1 input boolean size=1; reason output double size=1; r2 input boolean size=1; r3 input boolean size=1; r4 input boolean size=1; a1 input boolean size=1; a2 input boolean size=1; a3 input boolean size=1; a4 input boolean size=1
function reason = req_reject_reason(r1,r2,r3,r4,a1,a2,a3,a4)
%#codegen
raw = (r1 > 0.5) || (r2 > 0.5) || (r3 > 0.5) || (r4 > 0.5);
acc = (a1 > 0.5) || (a2 > 0.5) || (a3 > 0.5) || (a4 > 0.5);
if raw && ~acc
    reason = 1.0;
else
    reason = 0.0;
end

== matlab function E010A5_R3_E1_event_queue_alloc_40A_1A_20260701_085331/E010A5_PhaseOrderError ==
  data: a1 input boolean size=1; err output double size=1; a2 input boolean size=1; a3 input boolean size=1; a4 input boolean size=1; t input double size=1; t_step input double size=1
function err = phase_order_error(a1,a2,a3,a4,t,t_step)
%#codegen
persistent prev expected
if isempty(prev)
    prev = [false,false,false,false];
end
if isempty(expected)
    expected = 0.0;
end
acc = [a1,a2,a3,a4] > 0.5;
rise = acc & ~prev;
err = 0.0;
if t < t_step
    expected = 0.0;
else
    for idx = 1:4
        if rise(idx)
            if expected > 0.5 && double(idx) ~= expected
                err = 1.0;
            end
            expected = double(idx + 1);
            if expected > 4.0
                expected = 1.0;
            end
        end
    end
end
prev = acc;

== matlab function E010A5_R3_E1_event_queue_alloc_40A_1A_20260701_085331/E010A5_SevereDropDetector ==
  data: iload input double size=1; detected output double size=1; t input double size=1; threshold input double size=1
function detected = severe_drop_detector(iload,t,threshold)
%#codegen
persistent initial_load latched
if isempty(initial_load)
    initial_load = iload;
end
if isempty(latched)
    latched = false;
end
if t < 1.0e-9
    initial_load = iload;
    latched = false;
end
if (initial_load - iload) >= threshold
    latched = true;
end
detected = double(latched);

== matlab function E010A5_R3_E1_event_queue_alloc_40A_1A_20260701_085331/E010A5_TonActual1 ==
  data: qh input boolean size=1; Ton_actual output double size=1; t input double size=1
function Ton_actual = ton_actual_estimator(qh, t)
%#codegen
persistent q_prev t_rise last_width
if isempty(q_prev)
    q_prev = 0.0;
end
if isempty(t_rise)
    t_rise = 0.0;
end
if isempty(last_width)
    last_width = 0.0;
end
is_high = double(qh > 0.5);
if is_high > 0.5 && q_prev <= 0.5
    t_rise = t;
elseif is_high <= 0.5 && q_prev > 0.5
    last_width = max(0.0, t - t_rise);
end
Ton_actual = last_width;
q_prev = is_high;

== matlab function E010A5_R3_E1_event_queue_alloc_40A_1A_20260701_085331/E010A5_TonActual2 ==
  data: qh input boolean size=1; Ton_actual output double size=1; t input double size=1
function Ton_actual = ton_actual_estimator(qh, t)
%#codegen
persistent q_prev t_rise last_width
if isempty(q_prev)
    q_prev = 0.0;
end
if isempty(t_rise)
    t_rise = 0.0;
end
if isempty(last_width)
    last_width = 0.0;
end
is_high = double(qh > 0.5);
if is_high > 0.5 && q_prev <= 0.5
    t_rise = t;
elseif is_high <= 0.5 && q_prev > 0.5
    last_width = max(0.0, t - t_rise);
end
Ton_actual = last_width;
q_prev = is_high;

== matlab function E010A5_R3_E1_event_queue_alloc_40A_1A_20260701_085331/E010A5_TonActual3 ==
  data: qh input boolean size=1; Ton_actual output double size=1; t input double size=1
function Ton_actual = ton_actual_estimator(qh, t)
%#codegen
persistent q_prev t_rise last_width
if isempty(q_prev)
    q_prev = 0.0;
end
if isempty(t_rise)
    t_rise = 0.0;
end
if isempty(last_width)
    last_width = 0.0;
end
is_high = double(qh > 0.5);
if is_high > 0.5 && q_prev <= 0.5
    t_rise = t;
elseif is_high <= 0.5 && q_prev > 0.5
    last_width = max(0.0, t - t_rise);
end
Ton_actual = last_width;
q_prev = is_high;

== matlab function E010A5_R3_E1_event_queue_alloc_40A_1A_20260701_085331/E010A5_TonActual4 ==
  data: qh input boolean size=1; Ton_actual output double size=1; t input double size=1
function Ton_actual = ton_actual_estimator(qh, t)
%#codegen
persistent q_prev t_rise last_width
if isempty(q_prev)
    q_prev = 0.0;
end
if isempty(t_rise)
    t_rise = 0.0;
end
if isempty(last_width)
    last_width = 0.0;
end
is_high = double(qh > 0.5);
if is_high > 0.5 && q_prev <= 0.5
    t_rise = t;
elseif is_high <= 0.5 && q_prev > 0.5
    last_width = max(0.0, t - t_rise);
end
Ton_actual = last_width;
q_prev = is_high;

== matlab function E010A5_R3_E1_event_queue_alloc_40A_1A_20260701_085331/E010A5_ActiveHSPhase ==
  data: qh1 input boolean size=1; active_phase output double size=1; qh2 input boolean size=1; qh3 input boolean size=1; qh4 input boolean size=1
function active_phase = active_hs_phase(qh1,qh2,qh3,qh4)
%#codegen
qh = [qh1, qh2, qh3, qh4] > 0.5;
active_phase = 0.0;
for idx = 1:4
    if qh(idx)
        active_phase = double(idx);
        return;
    end
end

== matlab function E010A5_R3_E1_event_queue_alloc_40A_1A_20260701_085331/Ideal_Digital_IQCOT_Request/IQCOT_Event_Core ==
  data: e_v input double size=1; REQ_iqcot output double size=1; IL1 input double size=1; IL2 input double size=1; IL3 input double size=1; IL4 input double size=1; phase_idx input double size=1; tr_reset input double size=1; enable input double size=1; Ts_ctrl_in input double size=1; Lambda0_in input double size=1; Lambda_m2_in input double size=1; rho_cmd_in input double size=1; Ri_in input double size=1; Kvc_in input double size=1; Vc_bias_in input double size=1; kappa_cmd_in input double size=1; A_init_in input double size=1; A_lower_in input double size=1; A_upper_in input double size=1; A_iqcot output double size=1; Lambda_i output double size=1; h_iqcot output double size=1; IL_sel output double size=1; vc_ctrl output double size=1
function [REQ_iqcot,A_iqcot,Lambda_i,h_iqcot,IL_sel,vc_ctrl] = IQCOT_Event_Core(e_v,IL1,IL2,IL3,IL4,phase_idx,tr_reset,enable,Ts_ctrl_in,Lambda0_in,Lambda_m2_in,rho_cmd_in,Ri_in,Kvc_in,Vc_bias_in,kappa_cmd_in,A_init_in,A_lower_in,A_upper_in)
%#codegen
REQ_iqcot = 0.0;
A_iqcot = 0.0;
Lambda_i = 0.0;
h_iqcot = 0.0;
IL_sel = 0.0;
vc_ctrl = 0.0;
persistent Astate reset_prev phase_prev
if isempty(Astate)
    Astate = double(A_init_in);
end
if isempty(reset_prev)
    reset_prev = 0.0;
end
if isempty(phase_prev)
    phase_prev = 0.0;
end
p = floor(double(phase_idx));
p = mod(p, 4);
if p == 0
    IL_sel = IL1;
elseif p == 1
    IL_sel = IL2;
elseif p == 2
    IL_sel = IL3;
else
    IL_sel = IL4;
end
Ri_eff = Ri_in * exp(kappa_cmd_in);
vc_ctrl = Vc_bias_in + Kvc_in * e_v;
h_iqcot = vc_ctrl - Ri_eff * IL_sel;
Lambda_i = Lambda0_in * (1 + rho_cmd_in) + Lambda_m2_in * cos(pi * p);
if Lambda_i < eps
    Lambda_i = eps;
end
A_update = Astate + Ts_ctrl_in * h_iqcot;
if A_update < A_lower_in
    A_update = A_lower_in;
end
if A_update > A_upper_in
    A_update = A_upper_in;
end
REQ_iqcot = double((enable > 0.5) && (A_update >= Lambda_i));
A_iqcot = A_update;
reset_rise = (tr_reset > 0.5) && (reset_prev <= 0.5);
phase_change = (p ~= phase_prev);
if enable <= 0.5
    Astate = A_init_in;
elseif reset_rise || phase_change
    Astate = A_init_in;
else
    Astate = A_update;
end
reset_prev = double(tr_reset);
phase_prev = p;
